simulink model "DroneSim"  (R2024a)
settings: Solver=ode45  StartTime=0.0  StopTime=36000  RelTol=1e-3
values from neighbouring files (symbols this model uses):
  Initial = [0 0 0 0 0 0 0 0 0 0 0 0]    [RunMe.m]
  Ix = 0.0124    [RunMe.m]
  Iy = 0.0130    (= 0.013)    [RunMe.m]
  Iz = 0.0237    [RunMe.m]
  mass = 0.5    [RunMe.m]
  Ts = 0.1    [RunMe.m]    (also in testIfNewDynamicWork.m)
libraries: simulink_extras x3, sharedTrackingLibrary x1, mpclib x1
settings Model: Creator=liu12  LastModifiedBy=liu12

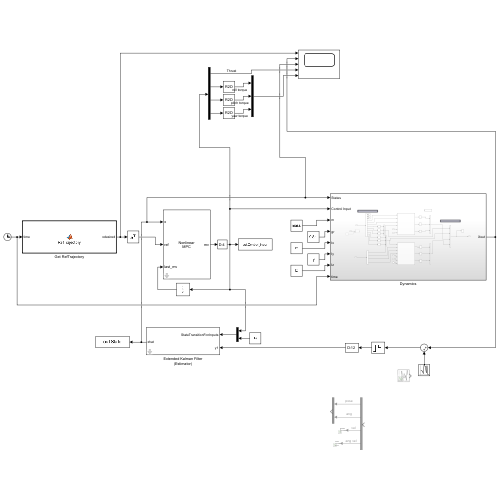
[thumbnail: Simulink's stored preview of the top-level diagram]
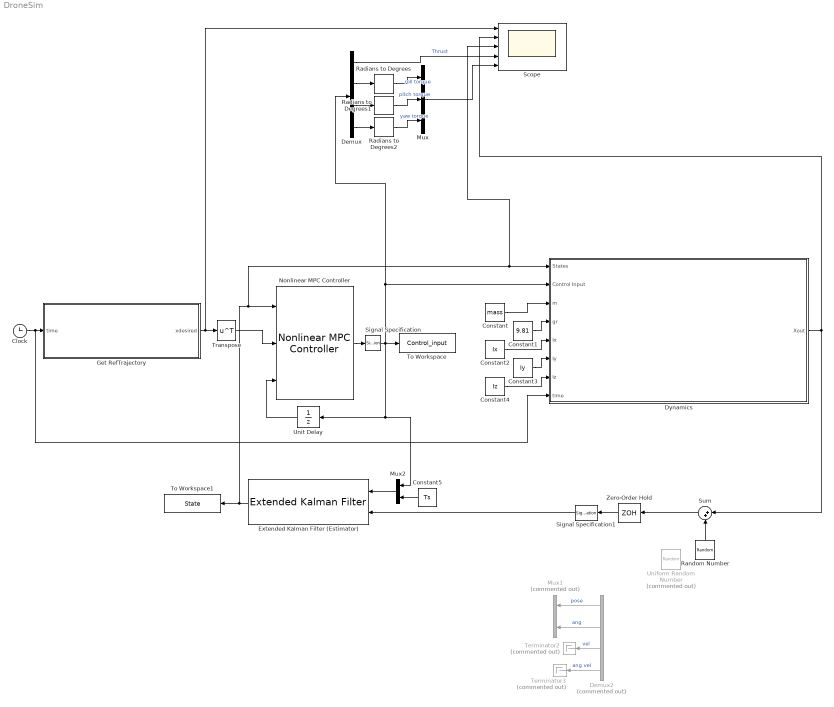
== system DroneSim ==
  Clock : Clock
  Constant : Constant  Value=mass
  Constant1 : Constant  Value=9.81
  Constant2 : Constant  Value=Ix
  Constant3 : Constant  Value=Iy
  Constant4 : Constant  Value=Iz
  Constant5 : Constant  Value=Ts
  Demux : Demux
  Demux2 : Demux  Commented=on
  Dynamics : Subsystem
  Extended Kalman Filter (Estimator) : sharedTrackingLibrary/Extended Kalman Filter  StateTransitionFcn=QuadrotorStateFcn  HasStateTransitionJacobianFcn=off  StateTransitionJacobianFcn=QuadrotorStateJacobianFcn  HasAdditiveProcessNoise=Additive  ProcessNoise=1e-4*eye(12)  HasTimeVaryingProcessNoise=off  HasStateTransitionFcnExtraArgument=1  InitialState=Initial  InitialStateCovariance=1e-4*eye(12)  MeasurementFcn1=QuadrotorMeasurementFcn  HasMeasurementJacobianFcn1=off  HasMeasurementEnablePort1=off  HasAdditiveMeasurementNoise1=Additive  MeasurementNoise1=1e-4*eye(12)  HasTimeVaryingMeasurementNoise1=off  HasMeasurementFcnExtraArgument1=0  HasMeasurementWrapping1=off  MeasurementFcn2=myMeasurementFcn  HasMeasurementJacobianFcn2=off  HasMeasurementEnablePort2=off  HasAdditiveMeasurementNoise2=Additive  MeasurementNoise2=1  HasTimeVaryingMeasurementNoise2=off  HasMeasurementFcnExtraArgument2=0  HasMeasurementWrapping2=off  MeasurementFcn3=myMeasurementFcn  HasMeasurementJacobianFcn3=off  HasMeasurementEnablePort3=off  HasAdditiveMeasurementNoise3=Additive  MeasurementNoise3=1  HasTimeVaryingMeasurementNoise3=off  HasMeasurementFcnExtraArgument3=0  HasMeasurementWrapping3=off  MeasurementFcn4=myMeasurementFcn  HasMeasurementJacobianFcn4=off  HasMeasurementEnablePort4=off  HasAdditiveMeasurementNoise4=Additive  MeasurementNoise4=1  HasTimeVaryingMeasurementNoise4=off  HasMeasurementFcnExtraArgument4=0  HasMeasurementWrapping4=off  MeasurementFcn5=myMeasurementFcn  HasMeasurementJacobianFcn5=off  HasMeasurementEnablePort5=off  HasAdditiveMeasurementNoise5=Additive  MeasurementNoise5=1  HasTimeVaryingMeasurementNoise5=off  HasMeasurementFcnExtraArgument5=0  HasMeasurementWrapping5=off  EnableMultirate=off  StateTransitionFcnSampleTime=1  MeasurementFcn1SampleTime=1  MeasurementFcn2SampleTime=1  MeasurementFcn3SampleTime=1  MeasurementFcn4SampleTime=1  MeasurementFcn5SampleTime=1  UseCurrentEstimator=on  OutputStateCovariance=off  DataType=double  SampleTime=Ts  NumberOfMeasurements=1
  Get RefTrajectory : MATLAB Function  TreatAsAtomicUnit=on
  Mux : Mux  Inputs=3
  Mux1 : Mux  Commented=on  Inputs=2
  Mux2 : Mux  Inputs=2
  Nonlinear MPC Controller : mpclib/Nonlinear MPC Controller  nlmpcobj=nlmpcobj  UseObjectTs=off  TsControl=Ts  UseMEX=off  md_enabled=off  mvtarget_enabled=off  param_enabled=off  cost_enabled=off  mvseq_enabled=off  stateseq_enabled=off  ovseq_enabled=off  slack_enabled=off  status_enabled=off  ov_min=off  ov_max=off  mv_min=off  mv_max=off  mvrate_min=off  mvrate_max=off  state_min=off  state_max=off  ov_weight=off  mv_weight=off  mvrate_weight=off  ecr_weight=off  nlp_initialize=off
  Radians to Degrees : simulink_extras/Transformations/Radians to Degrees
  Radians to Degrees1 : simulink_extras/Transformations/Radians to Degrees
  Radians to Degrees2 : simulink_extras/Transformations/Radians to Degrees
  Random Number : RandomNumber  Variance=0.001  SampleTime=Ts
  Scope : Scope  NumInputPorts=5
  Signal Specification : SignalSpecification  Dimensions=4
  Signal Specification1 : SignalSpecification  Dimensions=12
  Sum : Sum  Inputs=|++
  Terminator2 : Terminator  Commented=on
  Terminator3 : Terminator  Commented=on
  To Workspace : ToWorkspace  VariableName=Control_input  SaveFormat=Timeseries  SampleTime=-1
  To Workspace1 : ToWorkspace  VariableName=State  SaveFormat=Timeseries  SampleTime=-1
  Transpose : Math  Operator=transpose
  Uniform Random Number : UniformRandomNumber  Commented=on  Minimum=-0.01  Maximum=0.01  SampleTime=Ts
  Unit Delay : UnitDelay  SampleTime=-1  HasFrameUpgradeWarning=on
  Zero-Order Hold : ZeroOrderHold  SampleTime=Ts
  wires:
  Transpose/1 -> Nonlinear MPC Controller/2
  Constant/1 -> Dynamics/3(m)
  Constant1/1 -> Dynamics/4(gr)
  Constant2/1 -> Dynamics/5(Ix)
  Constant3/1 -> Dynamics/6(Iy)
  Constant4/1 -> Dynamics/7(Iz)
  Dynamics/1(Xout) -> Sum/1, Scope/2
  Clock/1 -> Dynamics/8(time), Get RefTrajectory/1(time)
  Get RefTrajectory/1(xdesired) -> Scope/1, Transpose/1
  Unit Delay/1 -> Nonlinear MPC Controller/3
  Demux/2 -> Radians to Degrees/1
  Demux/3 -> Radians to Degrees1/1
  Demux/4 -> Radians to Degrees2/1
  Demux/1 -> Scope/4  "Thrust"
  Radians to Degrees/1 -> Mux/1  "roll torque"
  Radians to Degrees1/1 -> Mux/2  "pitch torque"
  Radians to Degrees2/1 -> Mux/3  "yaw torque"
  Mux/1 -> Scope/5
  Sum/1 -> Zero-Order Hold/1
  Zero-Order Hold/1 -> Signal Specification1/1
  Signal Specification1/1 -> Extended Kalman Filter (Estimator)/2
  Nonlinear MPC Controller/1 -> Signal Specification/1
  Extended Kalman Filter (Estimator)/1 -> Scope/3, Dynamics/1(States), Nonlinear MPC Controller/1, To Workspace1/1
  Signal Specification/1 -> Demux/1, Dynamics/2(Control Input), To Workspace/1, Mux2/1, Unit Delay/1
  Demux2/4 -> Terminator3/1  "ang vel"
  Demux2/3 -> Terminator2/1  "vel"
  Demux2/2 -> Mux1/2  "ang"
  Demux2/1 -> Mux1/1  "pose"
  Mux2/1 -> Extended Kalman Filter (Estimator)/1
  Constant5/1 -> Mux2/2
  Random Number/1 -> Sum/2

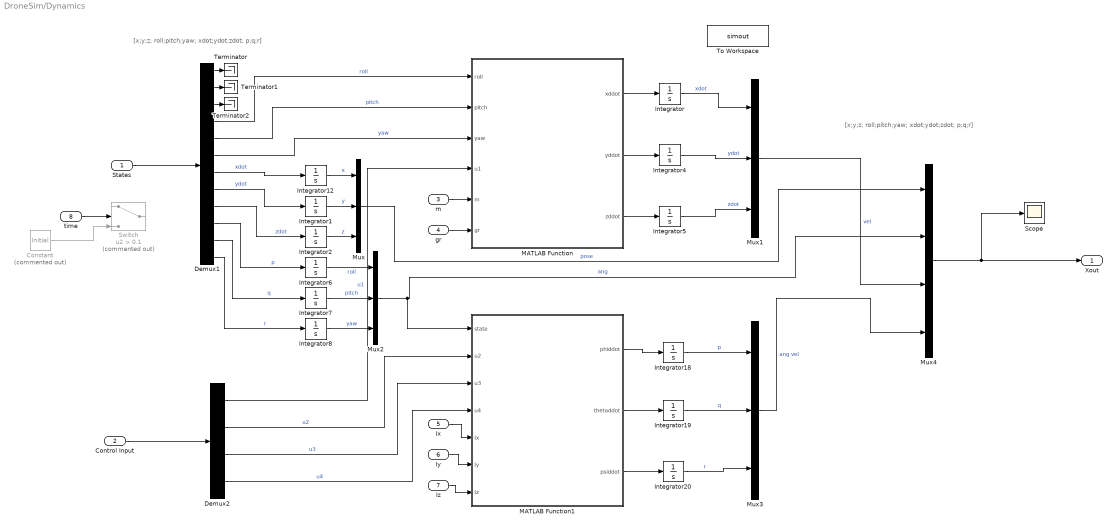
== system DroneSim/Dynamics ==
  note: [x;y;z; roll;pitch;yaw; xdot;ydot;zdot; p;q;r]
  note: [x;y;z; roll;pitch;yaw; xdot;ydot;zdot; p;q;r]
  States : Inport
  Control Input : Inport  Port=2
  m : Inport  Port=3
  gr : Inport  Port=4
  Ix : Inport  Port=5
  Iy : Inport  Port=6
  Iz : Inport  Port=7
  time : Inport  Port=8
  Constant : Constant  Commented=on  Value=Initial
  Demux1 : Demux  Outputs=12
  Demux2 : Demux
  Integrator{,1..2,4..8,12,18..20} (12 alike) : Integrator
  MATLAB Function : MATLAB Function  TreatAsAtomicUnit=on
  MATLAB Function1 : MATLAB Function  TreatAsAtomicUnit=on
  Mux{,1..3} (4 alike) : Mux  Inputs=3
  Mux4 : Mux
  Scope : Scope
  Switch : Switch  Commented=on  Criteria=u2 > Threshold  Threshold=0.1  SaturateOnIntegerOverflow=off  InputSameDT=off
  Terminator : Terminator
  Terminator1 : Terminator
  Terminator2 : Terminator
  To Workspace : ToWorkspace  VariableName=simout  SaveFormat=Timeseries  SampleTime=-1
  Xout : Outport
  wires:
  gr/1 -> MATLAB Function/6(gr)
  m/1 -> MATLAB Function/5(m)
  Demux2/1 -> MATLAB Function/4(u1)  "u1"
  Ix/1 -> MATLAB Function1/5(Ix)
  Iy/1 -> MATLAB Function1/6(Iy)
  Iz/1 -> MATLAB Function1/7(Iz)
  Demux2/2 -> MATLAB Function1/2(u2)  "u2"
  Demux2/3 -> MATLAB Function1/3(u3)  "u3"
  Demux2/4 -> MATLAB Function1/4(u4)  "u4"
  MATLAB Function/1(xddot) -> Integrator/1
  MATLAB Function/2(yddot) -> Integrator4/1
  MATLAB Function/3(zddot) -> Integrator5/1
  MATLAB Function1/2(thetaddot) -> Integrator19/1
  MATLAB Function1/1(phiddot) -> Integrator18/1
  MATLAB Function1/3(psiddot) -> Integrator20/1
  Demux1/4 -> MATLAB Function/1(roll)  "roll"
  Demux1/5 -> MATLAB Function/2(pitch)  "pitch"
  Demux1/6 -> MATLAB Function/3(yaw)  "yaw"
  Demux1/1 -> Terminator/1
  Demux1/2 -> Terminator1/1
  Demux1/3 -> Terminator2/1
  Demux1/7 -> Integrator12/1  "xdot"
  Demux1/8 -> Integrator1/1  "ydot"
  Demux1/9 -> Integrator2/1  "zdot"
  Control Input/1 -> Demux2/1
  Integrator12/1 -> Mux/1  "x"
  Integrator1/1 -> Mux/2  "y"
  Integrator2/1 -> Mux/3  "z"
  Integrator/1 -> Mux1/1  "xdot"
  Integrator4/1 -> Mux1/2  "ydot"
  Integrator5/1 -> Mux1/3  "zdot"
  Demux1/10 -> Integrator6/1  "p"
  Demux1/11 -> Integrator7/1  "q"
  Demux1/12 -> Integrator8/1  "r"
  Integrator7/1 -> Mux2/2  "pitch"
  Integrator6/1 -> Mux2/1  "roll"
  Integrator8/1 -> Mux2/3  "yaw"
  Integrator18/1 -> Mux3/1  "p"
  Integrator19/1 -> Mux3/2  "q"
  Integrator20/1 -> Mux3/3  "r"
  Mux4/1 -> Scope/1, Xout/1
  Mux/1 -> Mux4/1  "pose"
  Mux2/1 -> MATLAB Function1/1(state), Mux4/2  "ang"
  Mux1/1 -> Mux4/3  "vel"
  Mux3/1 -> Mux4/4  "ang vel"
  time/1 -> Switch/2
  Constant/1 -> Switch/3
  States/1 -> Demux1/1

== matlab function DroneSim/Dynamics/MATLAB Function1 ==
  data: state input; u2 input; phiddot output; u3 input; u4 input; Ix input; Iy input; thetaddot output; psiddot output; Iz input
function [phiddot, thetaddot, psiddot] = Angular_dynamics(state, u2, u3, u4, Ix, Iy, Iz)

%Inertia
% Ix = 0.0124; Iy = 0.0130; Iz = 0.0237;

phiddot = 0;
thetaddot = 0;
psiddot = 0;


p = state(1);
q = state(2);
r = state(3);

phiddot =  (q*r*((Iy-Iz)/Ix)) + (u2/Ix); % Roll Acceleration
thetaddot = (p*r*((Iz-Ix)/Iy)) + (u3/Iy); % Pitch Acceleration
psiddot =   (p*q*((Ix-Iy)/Iz)) + (u4/Iz); % Yaw Acceleration

end

== matlab function DroneSim/Dynamics/MATLAB Function ==
  data: roll input; xddot output; pitch input; yaw input; u1 input; m input; gr input; yddot output; zddot output
function [xddot, yddot, zddot] = nonlinear_Acc_dynamics(roll, pitch, yaw, u1, m, gr)

%Mass
% m = 0.5; % mass of copter [kg]

%Gravity
% gr = 9.81; %m/s^2

xddot = (1/m) * (-u1 * (cos(roll) * sin(pitch) * cos(yaw) + sin(roll) * sin(yaw))); % X-acceleration 
yddot = (1/m) * (-u1 * (cos(roll) * sin(pitch) * sin(yaw) - sin(roll) * cos(yaw))); % Y-acceleration
zddot = (1/m) * (u1 * cos(pitch) * cos(roll)) - gr; % Z-acceleration 

end

== matlab function DroneSim/Get RefTrajectory ==
  data: time input; xdesired output
function xdesired = RefTrajectory(time)
    xdesired = QuadrotorReferenceTrajectory(time);
end
